simulink model "lab2_model_bloczek"  (Simulink 7.5)
settings: Solver=ode45  StartTime=0.0  StopTime=20  RelTol=1e-3
values from neighbouring files (symbols this model uses):
  cpp = 1008    [skrypt.m]    (also in symulacja_dyn.m = cpp_; testerka.m)
  cpw = 4190    [skrypt.m]    (also in symulacja_dyn.m = cpw_; testerka.m)
  dFg = 0    [skrypt.m]    (also in symulacja_dyn.m = dFg_; testerka.m)
  dQt = dQt_    [symulacja_dyn.m]    (also in testerka.m = 0)
  dt = 5    [symulacja_dyn.m]
  dTgz = 0    [skrypt.m]    (also in symulacja_dyn.m = dTgz_; testerka.m)
  dTzew = dTzew_    [symulacja_dyn.m]    (also in testerka.m = 0)
  Fg_0 = Fg_n    (= 0.000243534167844)    [skrypt.m]    (also in symulacja_dyn.m = Fg_n)
  kg = Q_n/(Tgsr_n-Twew_n)    (= 400)    [skrypt.m]    (also in symulacja_dyn.m = Q_n/(Tgsr_n-Twew_n))
  kw = (Q_n-Qt_n)/(Twew_n-Tzew_n)    (= 500)    [skrypt.m]    (also in symulacja_dyn.m = (Q_n-Qt_0)/(Twew_n-Tzew_n))
  Qt_0 = 0    [symulacja_dyn.m]
  rop = 1.185    [skrypt.m]    (also in symulacja_dyn.m = rop_; testerka.m)
  row = 980    [skrypt.m]    (also in symulacja_dyn.m = row_; testerka.m)
  Tgsr_0 = Tgsr_n    [symulacja_dyn.m]
  Tgz_0 = Tgz_n    (= 90)    [skrypt.m]    (also in symulacja_dyn.m = Tgz_n)
  Twew_0 = Twew_n    (= 20)    [skrypt.m]    (also in symulacja_dyn.m = Twew_n)
  Tzew_0 = Tzew_n    (= -20)    [skrypt.m]    (also in symulacja_dyn.m = Tzew_n)
  Vg = 0.1    [skrypt.m]    (also in symulacja_dyn.m = Vg_; testerka.m)
  Vp = 75    [skrypt.m]    (also in symulacja_dyn.m = Vp_; testerka.m)
settings Model: Creator=LAB320-1537-User  LastModifiedBy=Spawek
settings DebuggingCC: FcnCallInpInsideContextMsg=Enable All

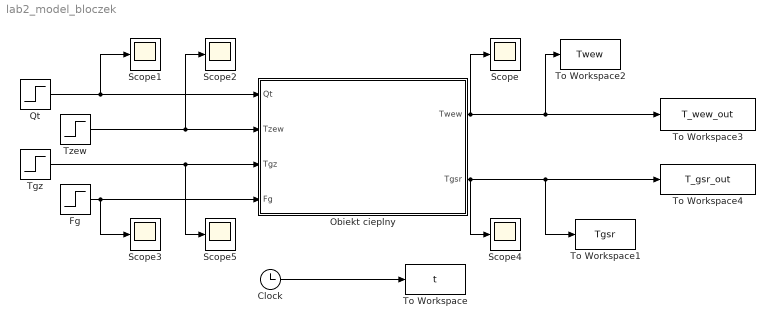
== system lab2_model_bloczek ==
  Clock : Clock
      settings: Decimation=10
  Fg : Step  Time=dt  Before=Fg_0  After=Fg_0+dFg  SampleTime=0
  Obiekt cieplny : Subsystem  mask{Vg=Vg, Vp=Vp, cpw=cpw, row=row, cpp=cpp, rop=rop, kg=kg, kw=kw, Twew_0=Twew_0, Tgsr_0=Tgsr_0}
      mask prompts: Vg "Objetosc grzejnika [m3]"; Vp "Objetosc pomieszczenia [m3]"; cpw "Cieplo wlasciwe cieczy"; row "Gestosc cieczy"; cpp "Cieplo wlasciwe powietrza"; rop "Gestosc powietrza"; kg "Wsp. przewodzenia grzejnika"; kw "Wsp. przewodzenia scian"; Twew_0 "Temp. pocz. wewnatrz"; Tgsr_0 "Temp. pocz. grzejnika"
  Qt : Step  Time=dt  Before=Qt_0  After=Qt_0+dQt  SampleTime=0
  Scope{,1..5} (6 alike) : Scope
      Scope settings: SaveName=ScopeData2
      Scope1 settings: SaveName=ScopeData3
      Scope3 settings: SaveName=ScopeData5
      Scope5 settings: SaveName=ScopeData4
  Tgz : Step  Time=dt  Before=Tgz_0  After=Tgz_0+dTgz  SampleTime=0
  To Workspace : ToWorkspace  VariableName=t  SampleTime=-1  SaveFormat=Array
  To Workspace1 : ToWorkspace  VariableName=Tgsr  SampleTime=-1  SaveFormat=Array
  To Workspace2 : ToWorkspace  VariableName=Twew  SampleTime=-1  SaveFormat=Array
  To Workspace3 : ToWorkspace  VariableName=T_wew_out  SampleTime=-1  SaveFormat=Structure With Time
  To Workspace4 : ToWorkspace  VariableName=T_gsr_out  SampleTime=-1  SaveFormat=Structure With Time
  Tzew : Step  Time=dt  Before=Tzew_0  After=Tzew_0+dTzew  SampleTime=0
  wires:
  Obiekt cieplny/2(Tgsr) -> Scope4/1, To Workspace1/1, To Workspace4/1
  Obiekt cieplny/1(Twew) -> Scope/1, To Workspace2/1, To Workspace3/1
  Qt/1 -> Obiekt cieplny/1(Qt), Scope1/1
  Tzew/1 -> Obiekt cieplny/2(Tzew), Scope2/1
  Tgz/1 -> Obiekt cieplny/3(Tgz), Scope5/1
  Fg/1 -> Obiekt cieplny/4(Fg), Scope3/1
  Clock/1 -> To Workspace/1

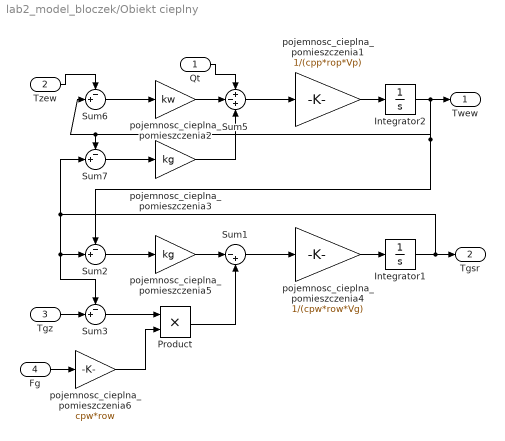
== system lab2_model_bloczek/Obiekt cieplny ==
  Qt : Inport
  Tzew : Inport  Port=2
  Tgz : Inport  Port=3
  Fg : Inport  Port=4
  Integrator1 : Integrator  InitialCondition=Tgsr_0
  Integrator2 : Integrator  InitialCondition=Twew_0
  Product : Product  RndMeth=Zero
  Sum1 : Sum  Inputs=|-+
  Sum{2..3,6..7} (4 alike) : Sum  Inputs=-+|
  Sum5 : Sum  Inputs=+-+
  pojemnosc_cieplna_pomieszczenia1 : Gain  Gain=1/(cpp*rop*Vp)
  pojemnosc_cieplna_pomieszczenia2 : Gain  Gain=kw
  pojemnosc_cieplna_pomieszczenia3 : Gain  Gain=kg
  pojemnosc_cieplna_pomieszczenia4 : Gain  Gain=1/(cpw*row*Vg)
  pojemnosc_cieplna_pomieszczenia5 : Gain  Gain=kg
  pojemnosc_cieplna_pomieszczenia6 : Gain  Gain=cpw*row
  Twew : Outport
  Tgsr : Outport  Port=2
  wires:
  pojemnosc_cieplna_pomieszczenia1/1 -> Integrator2/1
  Integrator2/1 -> Sum2/1, Sum7/1, Sum6/2, Twew/1
  Sum5/1 -> pojemnosc_cieplna_pomieszczenia1/1
  pojemnosc_cieplna_pomieszczenia2/1 -> Sum5/2
  pojemnosc_cieplna_pomieszczenia3/1 -> Sum5/3
  Sum6/1 -> pojemnosc_cieplna_pomieszczenia2/1
  Sum7/1 -> pojemnosc_cieplna_pomieszczenia3/1
  pojemnosc_cieplna_pomieszczenia4/1 -> Integrator1/1
  Integrator1/1 -> Sum2/2, Sum3/1, Sum7/2, Tgsr/1
  Sum1/1 -> pojemnosc_cieplna_pomieszczenia4/1
  Sum2/1 -> pojemnosc_cieplna_pomieszczenia5/1
  pojemnosc_cieplna_pomieszczenia5/1 -> Sum1/1
  pojemnosc_cieplna_pomieszczenia6/1 -> Product/2
  Sum3/1 -> Product/1
  Product/1 -> Sum1/2
  Qt/1 -> Sum5/1
  Tzew/1 -> Sum6/1
  Tgz/1 -> Sum3/2
  Fg/1 -> pojemnosc_cieplna_pomieszczenia6/1
